simulink model "FormaDirectaDoi"  (R2020b)
settings: Solver=VariableStepAuto  StartTime=0.0  StopTime=30.0  RelTol=1e-3
libraries: dspsnks4 x1, dspvision x1
settings Model: Creator=Nic  LastModifiedBy=Nic

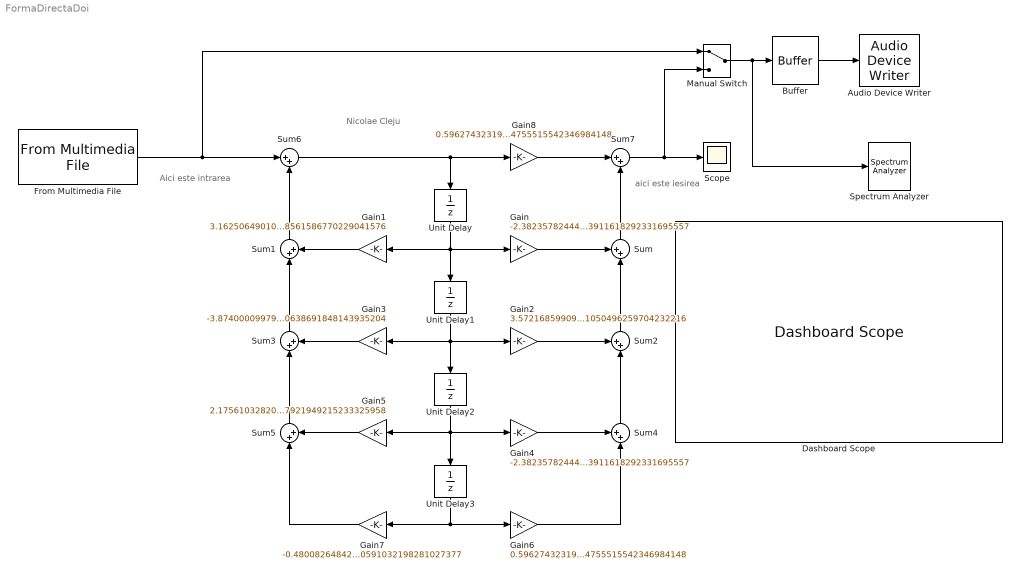
== system FormaDirectaDoi ==
  note: aici este iesirea
  note: Aici este intrarea
  note: Nicolae Cleju
  Audio Device Writer : dspsnks4/Audio Device Writer  Driver=DirectSound  Device=Default  InheritSampleRate=on  SampleRate=44100  BitDepth=16-bit integer  BufferSize=4096  NumBuffers=10  DefaultOutputChannelMapping=on  OutputChannelMapping=1:2  OutputNumUnderrunSamples=off  DriverIdx=1  DeviceWarnFlag=''
  Buffer : Buffer  N=1024  OutputFrames=off
  Dashboard Scope : DashboardScope
  From Multimedia File : dspvision/From Multimedia File  inputFilename=D:\2020_2021\PSS\Work\L04_5405\Labs_Sample.wav  readRange=[1 Inf]  loop=on  numPlays=inf  outputStreams=Audio only  videoDataType=single  audioDataType=double  inheritSampleTime=on  userDefinedSampleTime=1/30  noAudioOutput=off  isIntensityVideo=off  fourcc=RGB  colorVideoFormat=Separate color signals  outputEOF=off  dataOrg=Column-major  audioFrameSize=1  computeAudioFrameSize=off  outSamplingMode=Sample based
  Gain : Gain  Gain=-2.382357824447723260163911618292331695557
  Gain1 : Gain  Gain=3.162506490109901147178561586770229041576
  Gain2 : Gain  Gain=3.572168599097921948271050496259704232216
  Gain3 : Gain  Gain=-3.874000099792843876400638691848143935204
  Gain4 : Gain  Gain=-2.382357824447723260163911618292331695557
  Gain5 : Gain  Gain=2.175610328201987186957921949215233325958
  Gain6 : Gain  Gain=0.596274323195257638374755515542346984148
  Gain7 : Gain  Gain=-0.480082648426158498100591032198281027377
  Gain8 : Gain  Gain=0.596274323195257638374755515542346984148
  Manual Switch : ManualSwitch
  Scope : Scope
  Spectrum Analyzer : SpectrumAnalyzer
  Sum : Sum  Inputs=++|
  Sum{1,3,5..7} (5 alike) : Sum  Inputs=|++
  Sum2 : Sum  Inputs=++|
  Sum4 : Sum  Inputs=++|
  Unit Delay{,1..3} (4 alike) : UnitDelay  SampleTime=-1  HasFrameUpgradeWarning=on
  wires:
  Unit Delay/1 -> Unit Delay1/1, Gain/1, Gain1/1
  Gain/1 -> Sum/1
  Gain1/1 -> Sum1/2
  Unit Delay1/1 -> Unit Delay2/1, Gain2/1, Gain3/1
  Gain2/1 -> Sum2/1
  Gain3/1 -> Sum3/2
  Unit Delay2/1 -> Unit Delay3/1, Gain4/1, Gain5/1
  Gain4/1 -> Sum4/1
  Gain5/1 -> Sum5/2
  Unit Delay3/1 -> Gain6/1, Gain7/1
  Gain6/1 -> Sum4/2
  Gain7/1 -> Sum5/1
  Sum5/1 -> Sum3/1
  Sum3/1 -> Sum1/1
  Sum4/1 -> Sum2/2
  Sum2/1 -> Sum/2
  Sum1/1 -> Sum6/2
  Sum/1 -> Sum7/2
  Sum6/1 -> Unit Delay/1, Gain8/1
  Gain8/1 -> Sum7/1
  From Multimedia File/1 -> Manual Switch/1, Sum6/1
  Sum7/1 -> Manual Switch/2, Scope/1
  Buffer/1 -> Audio Device Writer/1
  Manual Switch/1 -> Spectrum Analyzer/1, Buffer/1
